simulink library "EasyGen3500_AIO_NGCHP_diesel_lib"  (Simulink 8.1)
settings: Solver=ode45  StartTime=0.0  StopTime=10.0  RelTol=1e-3
libraries: rtio_opalrt_common x6
settings Model: Creator=RE25624  LastModifiedBy=RE25624

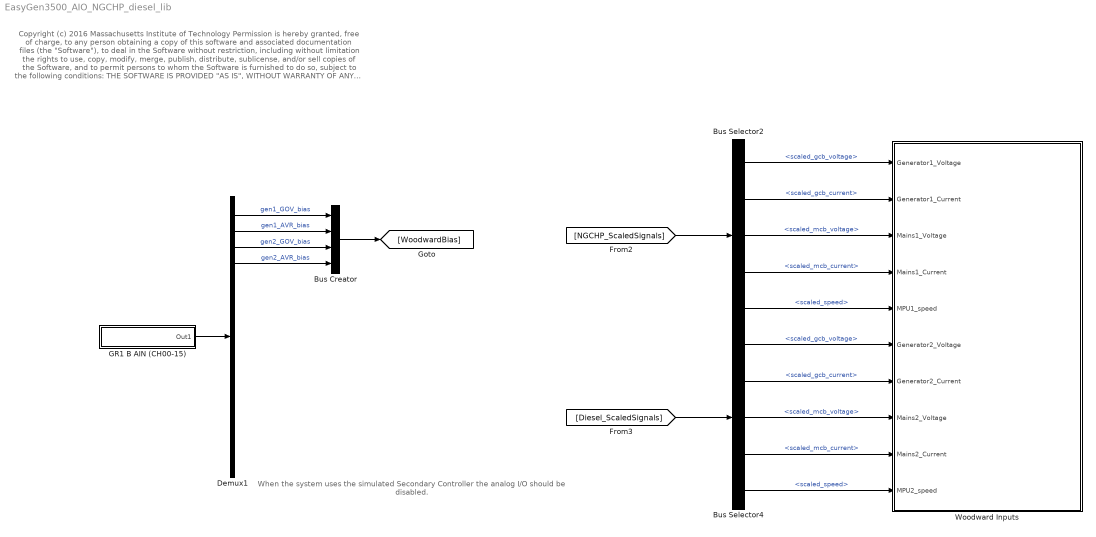
== system EasyGen3500_AIO_NGCHP_diesel_lib ==
  note: Copyright (c) 2016 Massachusetts Institute of Technology
      | Permission is hereby granted, free of charge, to any person obtaining a copy of this software and associated documentation files (the "Software"), to deal
      | in the Software without restriction, including without limitation the rights to use, copy, modify, merge, publish, distribute, sublicense, and/or sell copies of the
      | Software, and to permit persons to whom the Software is furnished to do so, subject to the following conditions:
      |
      | THE SOFTWARE IS PROVIDED "AS IS", WITHOUT WARRANTY OF ANY KIND, EXPRESS OR IMPLIED, INCLUDING BUT NOT LIMITED TO THE
      | WARRANTIES OF MERCHANTABILITY, FITNESS FOR A PARTICULAR PURPOSE AND NONINFRINGEMENT. IN NO EVENT SHALL THE AUTHORS
      | OR COPYRIGHT HOLDERS BE LIABLE FOR ANY CLAIM, DAMAGES OR OTHER LIABILITY, WHETHER IN AN ACTION OF CONTRACT, TORT OR
      | OTHERWISE, ARISING FROM, OUT OF OR IN CONNECTION WITH THE SOFTWARE OR THE USE OR OTHER DEALINGS IN THE SOFTWARE
  note: When the system uses the simulated
      | Secondary Controller the analog I/O
      | should be disabled.
  Bus Creator : BusCreator
  Bus Selector2 : BusSelector  OutputSignals=scaled_gcb_voltage,scaled_gcb_current,scaled_mcb_voltage,scaled_mcb_current,scaled_speed
  Bus Selector4 : BusSelector  OutputSignals=scaled_gcb_voltage,scaled_gcb_current,scaled_mcb_voltage,scaled_mcb_current,scaled_speed
  Demux1 : Demux  Outputs=16
  GR1 B AIN (CH00-15) : Subsystem
  Woodward Inputs : Subsystem
  wires:
  [NGCHP_ScaledSignals] -> Bus Selector2/1
  Bus Selector2/5 -> Woodward Inputs/5(MPU1_speed)  "<scaled_speed>"
  Bus Selector2/4 -> Woodward Inputs/4(Mains1_Current)  "<scaled_mcb_current>"
  Bus Selector2/3 -> Woodward Inputs/3(Mains1_Voltage)  "<scaled_mcb_voltage>"
  Bus Selector2/2 -> Woodward Inputs/2(Generator1_Current)  "<scaled_gcb_current>"
  Bus Selector2/1 -> Woodward Inputs/1(Generator1_Voltage)  "<scaled_gcb_voltage>"
  [Diesel_ScaledSignals] -> Bus Selector4/1
  Bus Selector4/1 -> Woodward Inputs/6(Generator2_Voltage)  "<scaled_gcb_voltage>"
  Bus Selector4/2 -> Woodward Inputs/7(Generator2_Current)  "<scaled_gcb_current>"
  Bus Selector4/3 -> Woodward Inputs/8(Mains2_Voltage)  "<scaled_mcb_voltage>"
  Bus Selector4/4 -> Woodward Inputs/9(Mains2_Current)  "<scaled_mcb_current>"
  Bus Selector4/5 -> Woodward Inputs/10(MPU2_speed)  "<scaled_speed>"
  GR1 B AIN (CH00-15)/1(Out1) -> Demux1/1
  Demux1/1 -> Bus Creator/1  "gen1_GOV_bias"
  Demux1/2 -> Bus Creator/2  "gen1_AVR_bias"
  Demux1/3 -> Bus Creator/3  "gen2_GOV_bias"
  Demux1/4 -> Bus Creator/4  "gen2_AVR_bias"
  Bus Creator/1 -> [WoodwardBias]

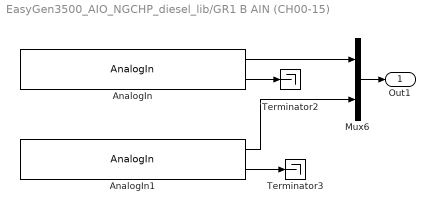
== system EasyGen3500_AIO_NGCHP_diesel_lib/GR1 B AIN (CH00-15) ==
  AnalogIn : rtio_opalrt_common/AnalogIn  CtrlName='OpCtrl'  portNb=1  FcnNos=Slot 1 Module B Subsection 1  size=16  maxcount=8  count=8  numchan=8  sampleTime=0
      settings: AttributesFormatString=%<CtrlName>
  AnalogIn1 : rtio_opalrt_common/AnalogIn  CtrlName='OpCtrl'  portNb=2  FcnNos=Slot 1 Module B Subsection 2  size=16  maxcount=8  count=8  numchan=8  sampleTime=0
      settings: AttributesFormatString=%<CtrlName>
  Mux6 : Mux  Inputs=2
  Terminator2 : Terminator
  Terminator3 : Terminator
  Out1 : Outport
  wires:
  Mux6/1 -> Out1/1
  AnalogIn1/2 -> Terminator3/1
  AnalogIn/2 -> Terminator2/1
  AnalogIn1/1 -> Mux6/2
  AnalogIn/1 -> Mux6/1

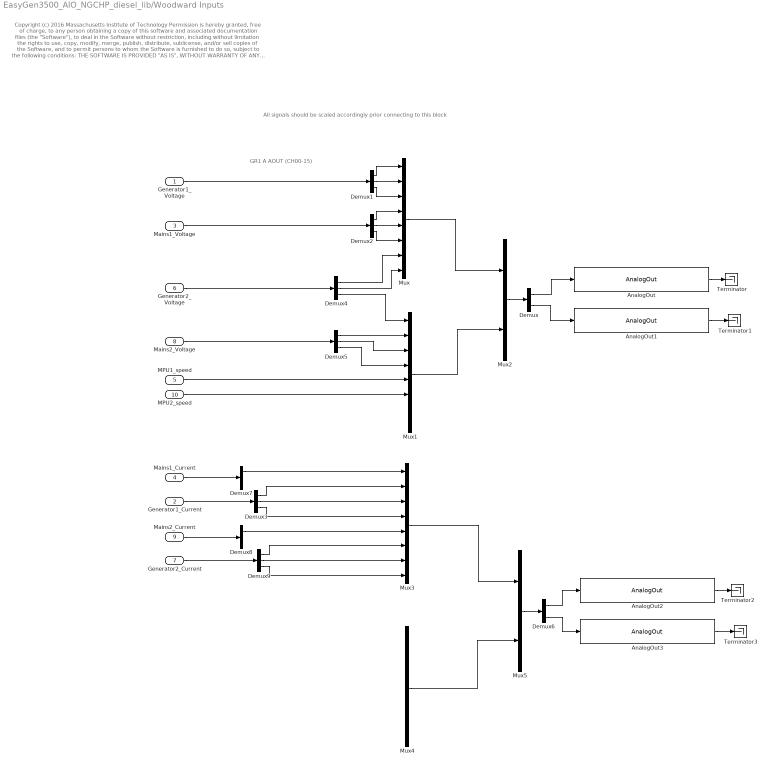
== system EasyGen3500_AIO_NGCHP_diesel_lib/Woodward Inputs ==
  note: Copyright (c) 2016 Massachusetts Institute of Technology
      | Permission is hereby granted, free of charge, to any person obtaining a copy of this software and associated documentation files (the "Software"), to deal
      | in the Software without restriction, including without limitation the rights to use, copy, modify, merge, publish, distribute, sublicense, and/or sell copies of the
      | Software, and to permit persons to whom the Software is furnished to do so, subject to the following conditions:
      |
      | THE SOFTWARE IS PROVIDED "AS IS", WITHOUT WARRANTY OF ANY KIND, EXPRESS OR IMPLIED, INCLUDING BUT NOT LIMITED TO THE
      | WARRANTIES OF MERCHANTABILITY, FITNESS FOR A PARTICULAR PURPOSE AND NONINFRINGEMENT. IN NO EVENT SHALL THE AUTHORS
      | OR COPYRIGHT HOLDERS BE LIABLE FOR ANY CLAIM, DAMAGES OR OTHER LIABILITY, WHETHER IN AN ACTION OF CONTRACT, TORT OR
      | OTHERWISE, ARISING FROM, OUT OF OR IN CONNECTION WITH THE SOFTWARE OR THE USE OR OTHER DEALINGS IN THE SOFTWARE
  note: GR1 A AOUT (CH00-15)
  note: All signals should be scaled accordingly prior connecting to this block
  Generator1_Voltage : Inport
  Generator1_Current : Inport  Port=2
  Mains1_Voltage : Inport  Port=3
  Mains1_Current : Inport  Port=4
  MPU1_speed : Inport  Port=5
  Generator2_Voltage : Inport  Port=6
  Generator2_Current : Inport  Port=7
  Mains2_Voltage : Inport  Port=8
  Mains2_Current : Inport  Port=9
  MPU2_speed : Inport  Port=10
  AnalogOut : rtio_opalrt_common/AnalogOut  CtrlName='OpCtrl'  portNb=1  FcnNos=Slot 1 Module A Subsection 1  size=16  maxcount=8  count=8  numchan=8  israngeinput=off  voltagerange=[-16 ... 16]  slot=0  side=0  mismatch=0  slotside=Slot_1_Module_A
      settings: AttributesFormatString=%<CtrlName>
  AnalogOut1 : rtio_opalrt_common/AnalogOut  CtrlName='OpCtrl'  portNb=2  FcnNos=Slot 1 Module A Subsection 2  size=16  maxcount=8  count=8  numchan=8  israngeinput=off  voltagerange=[-16 ... 16]  slot=0  side=0  mismatch=0  slotside=Slot_1_Module_A
      settings: AttributesFormatString=%<CtrlName>
  AnalogOut2 : rtio_opalrt_common/AnalogOut  CtrlName='OpCtrl'  portNb=3  FcnNos=Slot 2 Module A Subsection 1  size=16  maxcount=8  count=8  numchan=8  israngeinput=off  voltagerange=[-16 ... 16]  slot=1  side=0  mismatch=0  slotside=Slot_2_Module_A
      settings: AttributesFormatString=%<CtrlName>
  AnalogOut3 : rtio_opalrt_common/AnalogOut  CtrlName='OpCtrl'  portNb=4  FcnNos=Slot 2 Module A Subsection 2  size=16  maxcount=8  count=8  numchan=8  israngeinput=off  voltagerange=[-16 ... 16]  slot=1  side=0  mismatch=0  slotside=Slot_2_Module_A
      settings: AttributesFormatString=%<CtrlName>
  Demux : Demux  Outputs=2
  Demux{1..5,7..9} (8 alike) : Demux  Outputs=3
  Demux6 : Demux  Outputs=2
  Mux{,1,3..4} (4 alike) : Mux  Inputs=8
  Mux2 : Mux  Inputs=2
  Mux5 : Mux  Inputs=2
  Terminator{,1..3} (4 alike) : Terminator
  wires:
  Mains1_Voltage/1 -> Demux2/1
  Generator1_Voltage/1 -> Demux1/1
  Mux2/1 -> Demux/1
  Mux1/1 -> Mux2/2
  Mux/1 -> Mux2/1
  Demux/2 -> AnalogOut1/1
  Demux/1 -> AnalogOut/1
  AnalogOut1/1 -> Terminator1/1
  AnalogOut/1 -> Terminator/1
  Demux1/1 -> Mux/1
  Demux1/2 -> Mux/2
  Demux1/3 -> Mux/3
  Demux2/1 -> Mux/4
  Demux2/2 -> Mux/5
  Demux2/3 -> Mux/6
  MPU1_speed/1 -> Mux1/5
  Demux4/1 -> Mux/7
  Demux4/2 -> Mux/8
  Demux4/3 -> Mux1/1
  Demux5/1 -> Mux1/2
  Demux5/2 -> Mux1/3
  Demux5/3 -> Mux1/4
  Mux5/1 -> Demux6/1
  Mux4/1 -> Mux5/2
  Mux3/1 -> Mux5/1
  Demux6/2 -> AnalogOut3/1
  Demux6/1 -> AnalogOut2/1
  AnalogOut3/1 -> Terminator3/1
  AnalogOut2/1 -> Terminator2/1
  Generator1_Current/1 -> Demux3/1
  Demux3/1 -> Mux3/2
  Demux3/2 -> Mux3/3
  Demux3/3 -> Mux3/4
  Mains1_Current/1 -> Demux7/1
  Demux7/1 -> Mux3/1
  Mains2_Voltage/1 -> Demux5/1
  Generator2_Voltage/1 -> Demux4/1
  MPU2_speed/1 -> Mux1/6
  Mains2_Current/1 -> Demux8/1
  Demux8/1 -> Mux3/5
  Generator2_Current/1 -> Demux9/1
  Demux9/1 -> Mux3/6
  Demux9/2 -> Mux3/7
  Demux9/3 -> Mux3/8
